simulink library "sldvextractlib"  (Simulink 7.6)
settings: Solver=ode45  StartTime=0.0  StopTime=10.0  RelTol=1e-3
settings Model: Creator=The MathWorks Inc.

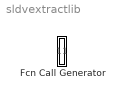
== system sldvextractlib ==
  Fcn Call Generator : Subsystem

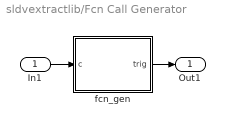
== system sldvextractlib/Fcn Call Generator ==
  In1 : Inport
  fcn_gen : Stateflow chart  TreatAsAtomicUnit=on
  Out1 : Outport
  wires:
  fcn_gen/1(trig) -> Out1/1
  In1/1 -> fcn_gen/1(c)

== stateflow chart Fcn Call Generator/fcn_gen ==
  (default) -> (junction 3) : [c] {trig;}
  data: c input boolean size=1
  events: trig output FUNCTION_CALL_EVENT
